simulink model "Combined_audioeffects"  (R2015a)
settings: Solver=ode45  StartTime=0.0  StopTime=10.0  RelTol=1e-3
libraries: dspsrcs4 x1, simulink x1, dspsigops x1, dspvision x1, dspsnks4 x1
settings Model: Creator=Meghna  LastModifiedBy=Meghna

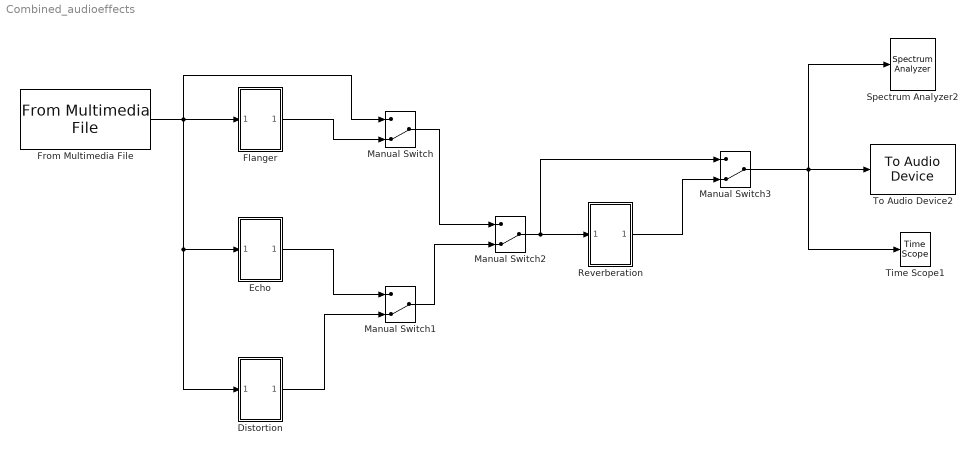
== system Combined_audioeffects ==
  "Distortion " : Subsystem
  "Echo " : Subsystem
  Flanger : Subsystem
  From Multimedia File : dspvision/From Multimedia File  inputFilename=speech_dft.mp3  loop=on  numPlays=inf  outputStreams=Audio only  videoDataType=single  audioDataType=double  inheritSampleTime=off  userDefinedSampleTime=1/30  noAudioOutput=off  isIntensityVideo=off  fourcc=RGB  colorVideoFormat=Separate color signals  outputEOF=off  dataOrg=Column-major  audioFrameSize=1000  computeAudioFrameSize=off  outSamplingMode=Sample based
  Manual Switch{,1..3} (4 alike) : ManualSwitch  CurrentSetting=0
  "Reverberation " : Subsystem
  Spectrum Analyzer2 : SpectrumAnalyzer
  Time Scope1 : TimeScope  DefaultConfigurationName=spbscopes.TimeScopeBlockCfg
  To Audio Device2 : dspsnks4/To Audio Device  deviceName=Default  inheritSampleRate=on  sampleRate=44100  deviceDatatype=Determine from input data type  autoBufferSize=on  bufferSize=4096  queueDuration=1.0  defaultOutputChannelMapping=on  outputChannelMapping=1:2  outputNumUnderrunSamples=off
  wires:
  "Echo "/1(Out1) -> Manual Switch1/1
  From Multimedia File/1 -> Manual Switch/1, "Distortion "/1(In1), "Echo "/1(In1), Flanger/1(In1)
  Manual Switch2/1 -> Manual Switch3/1, "Reverberation "/1(In1)
  Manual Switch/1 -> Manual Switch2/1
  Manual Switch1/1 -> Manual Switch2/2
  "Distortion "/1(Out1) -> Manual Switch1/2
  Flanger/1(Out1) -> Manual Switch/2
  "Reverberation "/1(Out1) -> Manual Switch3/2
  Manual Switch3/1 -> Time Scope1/1, To Audio Device2/1, Spectrum Analyzer2/1

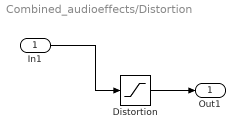
== system Combined_audioeffects/Distortion  ==
  In1 : Inport
  "Distortion " : Saturate
  Out1 : Outport
  wires:
  In1/1 -> "Distortion "/1
  "Distortion "/1 -> Out1/1

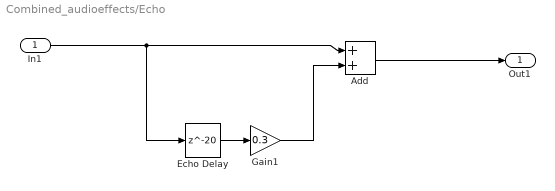
== system Combined_audioeffects/Echo  ==
  In1 : Inport
  Add : Sum
  Echo Delay : Delay  DelayLength=20  InitialCondition=0
  Gain1 : Gain  Gain=0.3
  Out1 : Outport
  wires:
  In1/1 -> Echo Delay/1, Add/1
  Add/1 -> Out1/1
  Echo Delay/1 -> Gain1/1
  Gain1/1 -> Add/2

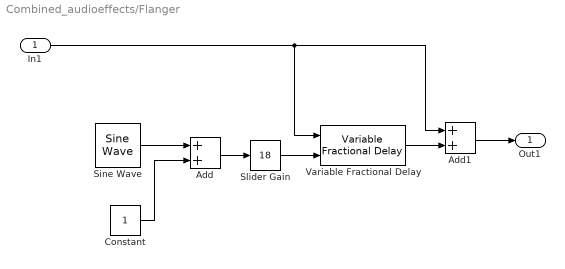
== system Combined_audioeffects/Flanger ==
  In1 : Inport
  Add : Sum
  Add1 : Sum
  Constant : Constant  SampleTime=1
  Sine Wave : dspsrcs4/Sine Wave  Amplitude=1  Frequency=100  Phase=0  SampleMode=Discrete  OutComplex=Real  CompMethod=Trigonometric fcn  TableSize=Speed  SampleTime=1  SamplesPerFrame=1  ResetState=Restart at time zero  dataType=double  wordLen=16  udDataType=sfix(16)  fracBitsMode=Best precision  numFracBits=15  OutDataTypeStr=double  LastOutDataTypeStr=double
  Slider Gain : simulink/Math Operations/Slider Gain  low=0  gain=18  high=36
  Variable Fractional Delay : dspsigops/Variable Fractional Delay  mode=OBSOLETE  modeActive=Linear  dmax=100  InputProcessing=Columns as channels (frame based)  L=4  FarrowL=4  R=10  alpha=1  ic=0  fallbackFIR=Clip to the minimum value necessary for centered kernel  fallbackFarrow=Clip to the minimum value necessary for centered kernel  noDFT=off  roundingMode=Zero  overflowMode=on
  Out1 : Outport
  wires:
  Sine Wave/1 -> Add/1
  Add/1 -> Slider Gain/1
  Slider Gain/1 -> Variable Fractional Delay/2
  In1/1 -> Add1/1, Variable Fractional Delay/1
  Constant/1 -> Add/2
  Add1/1 -> Out1/1
  Variable Fractional Delay/1 -> Add1/2

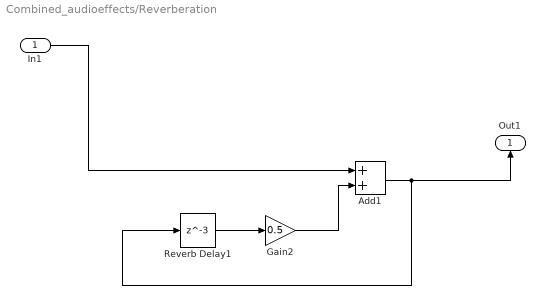
== system Combined_audioeffects/Reverberation  ==
  In1 : Inport
  Add1 : Sum
  Gain2 : Gain  Gain=0.5
  Reverb Delay1 : Delay  DelayLength=3  InitialCondition=0
  Out1 : Outport
  wires:
  In1/1 -> Add1/1
  Add1/1 -> Out1/1, Reverb Delay1/1
  Gain2/1 -> Add1/2
  Reverb Delay1/1 -> Gain2/1
